simulink model "OFDM0010"  (Simulink 7.7)
settings: Solver=ode45  StartTime=0.0  StopTime=0.08  RelTol=1e-3
undefined symbols (not defined in the file): get, i, rsgenpoly
libraries: dspobslib x46, dspindex x4, commsink2 x3, commutil2 x3, commchan3 x2, commdigbbndam3 x2, dspxfrm3 x2, commblkcod2 x2, commseqgen2 x2, commdigbbndpm3 x2, commrandsrc2 x1, dspsigops x1
Description:
  | This COFDM Simulation by
  | YangZhiguo
  |  .HuNan University at
  |  2011/05/21.
  | The teacher is
  |  xiaoyaoqiang !
  | Thanks to him!
  | This COFDM Simulation simulate Coded OFDM using
  | Reed-Solomon Channel Coding, over wireless multipath
  | fading channel, with 3 us maximal delay spread, 200 Hz
  | Doppler shift.
  | In this simulation I use QPSK, and Training Based
  | Channel Estimation, 11/15 RS Code, 2 Symbol Error
  | Correction
settings Model: Creator=Yangzhiguo  LastModifiedBy=yangzhiguo
settings SolverCC: MaxConsecutiveZCs=10
settings DataIOCC: SignalLoggingName=sigsOut
settings OptimizationCC: InitFltsAndDblsToZero=on
settings DebuggingCC: SaveWithParameterizedLinksMsg=none  SignalResolutionControl=TryResolveAllWithWarning  SolverPrmCheckMsg=none  MultiTaskDSMMsg=warning  MultiTaskCondExecSysMsg=none  StrictBusMsg=None
settings HardwareCC: TargetUnknown=on
settings RTWCC: IncludeERTFirstTime=on

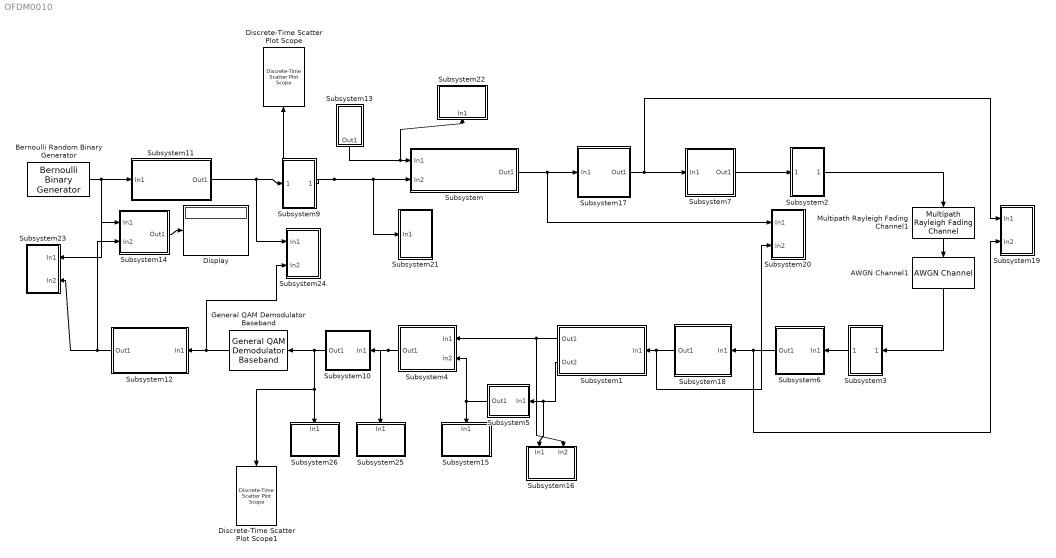
== system OFDM0010 ==
  AWGN Channel1 : commchan3/AWGN Channel  SystemSampleTime=-1  InputProcessing=Inherited (this choice will be removed - see release notes)  seed=32965  noiseMode="Signal to noise ratio  (SNR)"  EbNodB=10  EsNodB=28  SNRdB=-5  bitsPerSym=1  Ps=30/(5.5e5*11/15*2.4)*1.08  Tsym=80e-6  variance=1
  Bernoulli Random Binary Generator : commrandsrc2/Bernoulli Binary Generator  SystemSampleTime=-1  P=[0.5]  seed=9364248  Ts=16e-5/88/2  frameBased=on  sampPerFrame=88  orient=off  outDataType=double
  Discrete-Time Scatter Plot Scope : commsink2/Discrete-Time Scatter Plot Scope  Tag=ScatterPlot  SystemSampleTime=-1  sampPerSymb=1  offsetEye=0  numTraces=40  numNewFrames=40  LineMarkers=.  LineColors=b  fading=on  render=on  AxisGrid=on  xMin=-3.3  xMax=3.315  yMin=-3.3  yMax=3.315  inphaseLabel=In-phase Amplitude  quadratureLabel=Quadrature Amplitude  openScopeAtSimStart=on  FrameNumber=off  FigPos=get(0,'defaultfigureposition');  figTitle=Scatter Plot  numLinesMax=8  block_type_=scatter
  Discrete-Time Scatter Plot Scope1 : commsink2/Discrete-Time Scatter Plot Scope  Tag=ScatterPlot  SystemSampleTime=-1  sampPerSymb=1  offsetEye=0  numTraces=40  numNewFrames=40  LineMarkers=.  LineColors=b  fading=on  render=on  AxisGrid=on  xMin=-3.3  xMax=3.315  yMin=-3.3  yMax=3.315  inphaseLabel=In-phase Amplitude  quadratureLabel=Quadrature Amplitude  openScopeAtSimStart=on  FrameNumber=off  FigPos=get(0,'defaultfigureposition');  figTitle=Scatter Plot  numLinesMax=8  block_type_=scatter
  Display : Display
  General QAM Demodulator Baseband : commdigbbndam3/General QAM Demodulator Baseband  SigCon=[exp(2*pi*i*[0:15]/16)]  OutType=Bit  DecType=Hard decision  VarSource=Dialog  Variance=1  outDtypeBit=Inherit via internal rule  outDtype=Inherit via internal rule  roundingMode=Floor  overflowMode=Wrap  sigConstWordLen=16  accum1WordLen=32  accum1FracLen=30  prodInWordLen=32  prodInFracLen=30  prodOutWordLen=32  prodOutFracLen=30  accum2WordLen=32  accum2FracLen=30  accum3WordLen=32  accum3FracLen=30  nsiWordLen=32  nsiFracLen=30  invn0WordLen=16  invn0FracLen=8  outputWordLen=32  outputFracLen=30
  Multipath Rayleigh Fading Channel1 : commchan3/Multipath Rayleigh Fading Channel  SystemSampleTime=-1  maxDopplerShift=40  spectrumType=Jakes  sigmaGaussian=1/sqrt(2)  coeffRounded=[1 -1.72 0.785]  freqMinMaxRJakes=[0 1]  freqMinMaxAJakes=[0 1]  sigmaGaussian1=1/sqrt(2)  sigmaGaussian2=1/sqrt(2)  centerFreqGaussian1=0.0  centerFreqGaussian2=0.0  gainGaussian1=0.5  gainGaussian2=0.5  coeffBell=9  dopplerSpectrum=doppler.jakes  pathDelays=[0 2e-6]  avgPathGaindB=[0 -12]  normalizePathGains=on  seed=73  enableProbe=0  openVisAtStart=off  outPathGains=off  outDelay=off
  Subsystem : Subsystem
      mask Display: disp('OFDM Baseband\nModulator\ndan\nAdd Cyclic Prefix')
  Subsystem1 : Subsystem
      mask Display: disp('OFDM Baseband\nDemodulator\ndan \nRemove Cyclic prefix')
  Subsystem10 : Subsystem
      mask Display: disp('Remove\nZero')
  Subsystem11 : Subsystem
      mask Display: disp('RS(15,11) Encoder')
  Subsystem12 : Subsystem
      mask Display: disp('RS(15,11) Decoder')
  Subsystem13 : Subsystem
      mask Display: disp('Training')
  Subsystem14 : Subsystem
      mask Display: disp('SER\nCalculation')
  Subsystem15 : Subsystem
  Subsystem16 : Subsystem
  Subsystem17 : Subsystem
      mask Display: disp('Add\nCyclic Prefix')
  Subsystem18 : Subsystem
      mask Display: disp('Remove\nCyclic Prefix')
  Subsystem19 : Subsystem
  Subsystem2 : Subsystem
      mask Display: disp('P/S')
  Subsystem20 : Subsystem
  Subsystem21 : Subsystem
  Subsystem22 : Subsystem
  Subsystem23 : Subsystem
  Subsystem24 : Subsystem
  Subsystem25 : Subsystem
  Subsystem26 : Subsystem
  Subsystem3 : Subsystem
      mask Display: disp('S/P')
  Subsystem4 : Subsystem
      mask Display: disp('Channel\nCompensation')
  Subsystem5 : Subsystem
      mask Display: disp('Channel\nEstimator')
  Subsystem6 : Subsystem
      mask Display: disp('Training\nSeparation')
  Subsystem7 : Subsystem
      mask Display: disp('Training\nInsertion')
  Subsystem9 : Subsystem
      mask Display: disp('16QAM')
  wires:
  Bernoulli Random Binary Generator/1 -> Subsystem14/1(In1), Subsystem11/1(In1), Subsystem23/1(In1)
  Subsystem9/1(Out1) -> Subsystem/2(In2), Subsystem21/1(In1), Discrete-Time Scatter Plot Scope/1
  Subsystem13/1(Out1) -> Subsystem/1(In1), Subsystem22/1(In1)
  Subsystem12/1(Out1) -> Subsystem14/2(In2), Subsystem23/2(In2)
  Subsystem/1(Out1) -> Subsystem17/1(In1), Subsystem20/1(In1)
  Subsystem7/1(Out1) -> Subsystem2/1(In1)
  Subsystem6/1(Out1) -> Subsystem18/1(In1), Subsystem19/2(In2)
  Subsystem14/1(Out1) -> Display/1
  Subsystem3/1(Out1) -> Subsystem6/1(In1)
  Subsystem2/1(Out1) -> Multipath Rayleigh Fading Channel1/1
  Subsystem10/1(Out1) -> Subsystem26/1(In1), Discrete-Time Scatter Plot Scope1/1, General QAM Demodulator Baseband/1
  Multipath Rayleigh Fading Channel1/1 -> AWGN Channel1/1
  AWGN Channel1/1 -> Subsystem3/1(In1)
  Subsystem4/1(Out1) -> Subsystem10/1(In1), Subsystem25/1(In1)
  Subsystem1/1(Out1) -> Subsystem4/1(In1), Subsystem16/2(In2)
  Subsystem5/1(Out1) -> Subsystem4/2(In2), Subsystem15/1(In1)
  Subsystem1/2(Out2) -> Subsystem5/1(In1), Subsystem16/1(In1)
  Subsystem17/1(Out1) -> Subsystem7/1(In1), Subsystem19/1(In1)
  Subsystem18/1(Out1) -> Subsystem1/1(In1), Subsystem20/2(In2)
  General QAM Demodulator Baseband/1 -> Subsystem12/1(In1), Subsystem24/2(In2)
  Subsystem11/1(Out1) -> Subsystem24/1(In1), Subsystem9/1(In1)

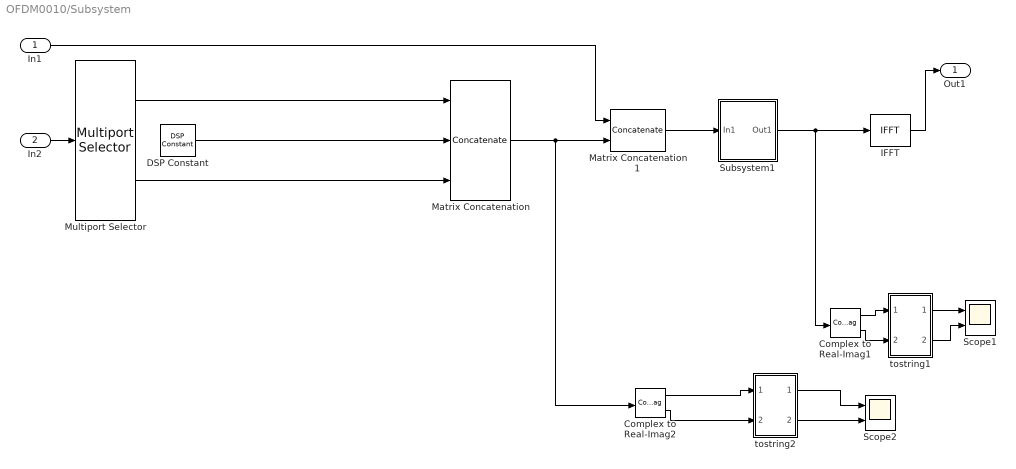
== system OFDM0010/Subsystem ==
  In1 : Inport
  In2 : Inport  Port=2
  Complex to Real-Imag1 : ComplexToRealImag
  Complex to Real-Imag2 : ComplexToRealImag
  DSP Constant : dspobslib/DSP Constant  SystemSampleTime=-1  Value=0  SampleMode=Discrete  discreteOutput=Frame-based  continuousOutput=Sample-based  sampTime=16e-5/2  framePeriod=16e-5/2  dataType=Inherit from 'Constant value'  isSigned=on  wordLen=16  udDataType=sfix(16)  fracBitsMode=Best precision  numFracBits=15  InterpretAs1D=off  Ts=16e-5/2  FramebasedOutput=on
  IFFT : dspxfrm3/IFFT  CompMethod=Table lookup  TableOpt=HYBRID  TableOptActive=Speed  BitRevOrder=off  cs_in=off  SkipNorm=on  InheritFFTLength=on  FFTLength=64  mode=Real  outSamplingMode=Frame based  RowConvenienceOn=on  firstCoeffDataTypeStr=Inherit: Same word length as input  firstCoeffLastDataTypeStr=Inherit: Same word length as input  outputMin=[]  outputMax=[]  roundingMode=Floor  overflowMode=off
  Matrix Concatenation : Concatenate  NumInputs=3  Mode=Multidimensional array
  Matrix Concatenation1 : Concatenate  Mode=Multidimensional array  ConcatenateDimension=2
  Multiport Selector : dspindex/Multiport Selector  rowsOrCols=Rows  idxCellArray={1:15,16:30}  idxErrMode=Clip Index
  Scope1 : Scope  NumInputPorts=2
      settings: YMin=-5~-5  YMax=5~5  SaveName=ScopeData5
  Scope2 : Scope  NumInputPorts=2
      settings: YMin=-5~-5  YMax=5~5  SaveName=ScopeData6
  Subsystem1 : Subsystem
      mask Display: disp('Zero Pad')
  tostring1 : Subsystem
  tostring2 : Subsystem
  Out1 : Outport
  wires:
  IFFT/1 -> Out1/1
  Multiport Selector/1 -> Matrix Concatenation/1
  Multiport Selector/2 -> Matrix Concatenation/3
  DSP Constant/1 -> Matrix Concatenation/2
  Subsystem1/1(Out1) -> IFFT/1, Complex to Real-Imag1/1
  In2/1 -> Multiport Selector/1
  Matrix Concatenation1/1 -> Subsystem1/1(In1)
  Matrix Concatenation/1 -> Matrix Concatenation1/2, Complex to Real-Imag2/1
  In1/1 -> Matrix Concatenation1/1
  Complex to Real-Imag1/1 -> tostring1/1(In1)
  Complex to Real-Imag1/2 -> tostring1/2(In2)
  tostring1/1(Out1) -> Scope1/1
  tostring1/2(Out2) -> Scope1/2
  Complex to Real-Imag2/1 -> tostring2/1(In1)
  Complex to Real-Imag2/2 -> tostring2/2(In2)
  tostring2/1(Out1) -> Scope2/1
  tostring2/2(Out2) -> Scope2/2

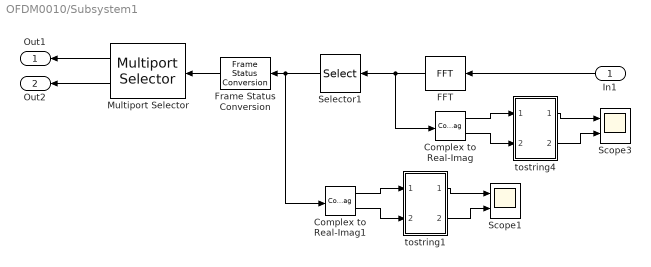
== system OFDM0010/Subsystem1 ==
  In1 : Inport
  Complex to Real-Imag : ComplexToRealImag
  Complex to Real-Imag1 : ComplexToRealImag
  FFT : dspxfrm3/FFT  CompMethod=Table lookup  TableOpt=HYBRID  TableOptActive=Speed  BitRevOrder=off  InheritFFTLength=on  FFTLength=64  RowConvenienceOn=on  SkipNorm=off  firstCoeffDataTypeStr=Inherit: Same word length as input  firstCoeffLastDataTypeStr=Inherit: Same word length as input  outputMin=[]  outputMax=[]  roundingMode=Floor  overflowMode=off
  Frame Status Conversion : dspobslib/Frame Status Conversion  SystemSampleTime=-1  growRefPort=off  outframe=Frame-based
  Multiport Selector : dspindex/Multiport Selector  rowsOrCols=Columns  idxCellArray={1,2}  idxErrMode=Clip Index
  Scope1 : Scope  NumInputPorts=2
      settings: YMin=-5~-5  YMax=5~5  SaveName=ScopeData9
  Scope3 : Scope  NumInputPorts=2
      settings: YMin=-5~-5  YMax=5~5  SaveName=ScopeData8
  Selector1 : Selector  NumberOfDimensions=2  InputPortWidth=64  IndexOptions=Index vector (dialog),Select all  Indices=[50:64,1:16],-1  OutputSizes=1
  tostring1 : Subsystem
  tostring4 : Subsystem
  Out1 : Outport
  Out2 : Outport  Port=2
  wires:
  FFT/1 -> Selector1/1, Complex to Real-Imag/1
  Selector1/1 -> Frame Status Conversion/1, Complex to Real-Imag1/1
  In1/1 -> FFT/1
  Frame Status Conversion/1 -> Multiport Selector/1
  Multiport Selector/1 -> Out1/1
  Multiport Selector/2 -> Out2/1
  Complex to Real-Imag/1 -> tostring4/1(In1)
  Complex to Real-Imag/2 -> tostring4/2(In2)
  tostring4/1(Out1) -> Scope3/1
  tostring4/2(Out2) -> Scope3/2
  Complex to Real-Imag1/1 -> tostring1/1(In1)
  Complex to Real-Imag1/2 -> tostring1/2(In2)
  tostring1/1(Out1) -> Scope1/1
  tostring1/2(Out2) -> Scope1/2

== system OFDM0010/Subsystem10 ==
  In1 : Inport
  Selector2 : Selector  NumberOfDimensions=2  InputPortWidth=31  IndexOptions=Index vector (dialog),Select all  Indices=[1:15,17:31],-1  OutputSizes=1
  Out1 : Outport
  wires:
  Selector2/1 -> Out1/1
  In1/1 -> Selector2/1

== system OFDM0010/Subsystem11 ==
  In1 : Inport
  Binary-Input RS Encoder : commblkcod2/Binary-Input RS Encoder  SystemSampleTime=-1  n=15  k=11  specPrimPoly=off  prPoly=[1 0 1 1]  specGenPoly=off  genPoly=rsgenpoly(7,3)  specPuncture=off  punctVec=[ones(2,1); zeros(2,1)]  outDType=Same as input
  Out1 : Outport
  wires:
  In1/1 -> Binary-Input RS Encoder/1
  Binary-Input RS Encoder/1 -> Out1/1

== system OFDM0010/Subsystem12 ==
  In1 : Inport
  Binary-Output RS Decoder : commblkcod2/Binary-Output RS Decoder  SystemSampleTime=-1  n=15  k=11  specPrimPoly=off  prPoly=[1 0 1 1]  specGenPoly=off  genPoly=rsgenpoly(7,3)  specPuncture=off  punctVec=[ones(2,1); zeros(2,1)]  specErasurePort=off  showNumErr=on  outDType=Same as input
  Terminator : Terminator
  Out1 : Outport
  wires:
  Binary-Output RS Decoder/2 -> Terminator/1
  Binary-Output RS Decoder/1 -> Out1/1
  In1/1 -> Binary-Output RS Decoder/1

== system OFDM0010/Subsystem13 ==
  PN Sequence Generator : commseqgen2/PN Sequence Generator  poly=[1 0 0 0 0 1 1]  ini_sta=[0 0 0 0 0 1]  outBitMaskSource=Dialog parameter  shift=0  outVarSiz=off  maxOutSizeMode=Dialog parameter  maxOutSize=[10 1]  Ts=16e-5/2/31  frameBased=on  sampPerFrame=31  reset=off  bitPackedOutputs=off  outDataType=double  numPackedBits=8  bitPackDataSigned=off  bitPackedOutDType=double
  Unipolar to Bipolar Converter : commutil2/Unipolar to Bipolar Converter  SystemSampleTime=-1  M=2  polarity=Positive  dataType=Inherit via internal rule
  Out1 : Outport
  wires:
  PN Sequence Generator/1 -> Unipolar to Bipolar Converter/1
  Unipolar to Bipolar Converter/1 -> Out1/1

== system OFDM0010/Subsystem14 ==
  In1 : Inport
  In2 : Inport  Port=2
  Error Rate Calculation : commsink2/Error Rate Calculation  N=44  st_delay=0  cp_mode=Entire frame  subframe=[]  PMode=Port  WsName=ErrorVec  RsMode2=off  stop=off  numErr=inf  maxBits=2e4
  QPSK Modulator Baseband : commdigbbndpm3/QPSK Modulator Baseband  SystemSampleTime=-1  InType=Bit  Enc=Binary  Ph=pi/4  outDtype=double  outWordLen=16  outUDDataType=sfix(16)  outFracLenMode=Best precision  outFracLen=15
  QPSK Modulator Baseband1 : commdigbbndpm3/QPSK Modulator Baseband  SystemSampleTime=-1  InType=Bit  Enc=Binary  Ph=pi/4  outDtype=double  outWordLen=16  outUDDataType=sfix(16)  outFracLenMode=Best precision  outFracLen=15
  Out1 : Outport
  wires:
  QPSK Modulator Baseband/1 -> Error Rate Calculation/1
  QPSK Modulator Baseband1/1 -> Error Rate Calculation/2
  In1/1 -> QPSK Modulator Baseband/1
  Error Rate Calculation/1 -> Out1/1
  In2/1 -> QPSK Modulator Baseband1/1

== system OFDM0010/Subsystem15 ==
  In1 : Inport
  Complex to Real-Imag7 : ComplexToRealImag
  Scope7 : Scope  NumInputPorts=2
      settings: YMin=-5~-5  YMax=5~5  SaveName=ScopeData11
  tostring9 : Subsystem
  wires:
  Complex to Real-Imag7/1 -> tostring9/1(In1)
  Complex to Real-Imag7/2 -> tostring9/2(In2)
  tostring9/1(Out1) -> Scope7/1
  tostring9/2(Out2) -> Scope7/2
  In1/1 -> Complex to Real-Imag7/1

== system OFDM0010/Subsystem16 ==
  In1 : Inport
  In2 : Inport  Port=2
  Complex to Real-Imag5 : ComplexToRealImag
  Complex to Real-Imag6 : ComplexToRealImag
  Scope6 : Scope  NumInputPorts=4
      settings: YMin=-5~-5~-5~-5  YMax=5~5~5~5  SaveName=ScopeData10
  tostring8 : Subsystem
  wires:
  tostring8/1(Out1) -> Scope6/1
  tostring8/2(Out2) -> Scope6/2
  Complex to Real-Imag5/1 -> tostring8/1(In1)
  Complex to Real-Imag5/2 -> tostring8/2(In2)
  Complex to Real-Imag6/1 -> tostring8/3(In3)
  Complex to Real-Imag6/2 -> tostring8/4(In4)
  tostring8/3(Out3) -> Scope6/3
  tostring8/4(Out4) -> Scope6/4
  In1/1 -> Complex to Real-Imag5/1
  In2/1 -> Complex to Real-Imag6/1

== system OFDM0010/Subsystem17 ==
  In1 : Inport
  Selector3 : Selector  NumberOfDimensions=2  InputPortWidth=64  IndexOptions=Index vector (dialog),Select all  Indices=[39:64,1:64],-1  OutputSizes=1
  Out1 : Outport
  wires:
  Selector3/1 -> Out1/1
  In1/1 -> Selector3/1

== system OFDM0010/Subsystem18 ==
  In1 : Inport
  Selector4 : Selector  NumberOfDimensions=2  InputPortWidth=78  IndexOptions=Index vector (dialog),Select all  Indices=[27:90],-1  OutputSizes=1
  Out1 : Outport
  wires:
  Selector4/1 -> Out1/1
  In1/1 -> Selector4/1

== system OFDM0010/Subsystem19 ==
  In1 : Inport
  In2 : Inport  Port=2
  Complex to Real-Imag1 : ComplexToRealImag
  Complex to Real-Imag2 : ComplexToRealImag
  Scope4 : Scope  NumInputPorts=4
      settings: YMin=-5~-5~-5~-5  YMax=5~5~5~5  SaveName=ScopeData7
  tostring5 : Subsystem
  tostring6 : Subsystem
  wires:
  Complex to Real-Imag1/1 -> tostring5/1(In1)
  Complex to Real-Imag1/2 -> tostring5/2(In2)
  tostring5/1(Out1) -> Scope4/1
  Complex to Real-Imag2/1 -> tostring6/1(In1)
  Complex to Real-Imag2/2 -> tostring6/2(In2)
  tostring6/1(Out1) -> Scope4/2
  tostring5/2(Out2) -> Scope4/3
  tostring6/2(Out2) -> Scope4/4
  In1/1 -> Complex to Real-Imag1/1
  In2/1 -> Complex to Real-Imag2/1

== system OFDM0010/Subsystem2 ==
  In1 : Inport
  Unbuffer3 : Unbuffer
  Out1 : Outport
  wires:
  In1/1 -> Unbuffer3/1
  Unbuffer3/1 -> Out1/1

== system OFDM0010/Subsystem20 ==
  In1 : Inport
  In2 : Inport  Port=2
  Complex to Real-Imag3 : ComplexToRealImag
  Complex to Real-Imag4 : ComplexToRealImag
  Scope5 : Scope  NumInputPorts=4
      settings: YMin=-5~-5~-5~-5  YMax=5~5~5~5  SaveName=ScopeData4
  tostring7 : Subsystem
  wires:
  Complex to Real-Imag3/1 -> tostring7/1(In1)
  Complex to Real-Imag3/2 -> tostring7/2(In2)
  tostring7/1(Out1) -> Scope5/1
  Complex to Real-Imag4/1 -> tostring7/3(In3)
  Complex to Real-Imag4/2 -> tostring7/4(In4)
  tostring7/3(Out3) -> Scope5/2
  tostring7/2(Out2) -> Scope5/3
  tostring7/4(Out4) -> Scope5/4
  In1/1 -> Complex to Real-Imag3/1
  In2/1 -> Complex to Real-Imag4/1

== system OFDM0010/Subsystem21 ==
  In1 : Inport
  Complex to Real-Imag : ComplexToRealImag
  Scope3 : Scope  NumInputPorts=2
      settings: YMin=-5~-5  YMax=5~5  SaveName=ScopeData3
  tostring4 : Subsystem
  wires:
  Complex to Real-Imag/1 -> tostring4/1(In1)
  Complex to Real-Imag/2 -> tostring4/2(In2)
  tostring4/1(Out1) -> Scope3/1
  tostring4/2(Out2) -> Scope3/2
  In1/1 -> Complex to Real-Imag/1

== system OFDM0010/Subsystem22 ==
  In1 : Inport
  Scope2 : Scope
      settings: SaveName=ScopeData2
  tostring3 : Subsystem
  wires:
  tostring3/1(Out1) -> Scope2/1
  In1/1 -> tostring3/1(In1)

== system OFDM0010/Subsystem23 ==
  In1 : Inport
  In2 : Inport  Port=2
  Scope : Scope  NumInputPorts=2
      settings: YMin=-5~-5  YMax=5~5
  tostring : Subsystem
  tostring1 : Subsystem
  wires:
  tostring/1(Out1) -> Scope/1
  tostring1/1(Out1) -> Scope/2
  In1/1 -> tostring/1(In1)
  In2/1 -> tostring1/1(In1)

== system OFDM0010/Subsystem24 ==
  In1 : Inport
  In2 : Inport  Port=2
  Scope1 : Scope  NumInputPorts=2
      settings: YMin=-5~-5  YMax=5~5
  tostring2 : Subsystem
  wires:
  tostring2/1(Out1) -> Scope1/1
  tostring2/2(Out2) -> Scope1/2
  In1/1 -> tostring2/1(In1)
  In2/1 -> tostring2/2(In2)

== system OFDM0010/Subsystem25 ==
  In1 : Inport
  Complex to Real-Imag7 : ComplexToRealImag
  Scope7 : Scope  NumInputPorts=2
      settings: YMin=-5~-5  YMax=5~5  SaveName=ScopeData11
  tostring9 : Subsystem
  wires:
  Complex to Real-Imag7/1 -> tostring9/1(In1)
  Complex to Real-Imag7/2 -> tostring9/2(In2)
  tostring9/1(Out1) -> Scope7/1
  tostring9/2(Out2) -> Scope7/2
  In1/1 -> Complex to Real-Imag7/1

== system OFDM0010/Subsystem26 ==
  In1 : Inport
  Complex to Real-Imag7 : ComplexToRealImag
  Scope7 : Scope  NumInputPorts=2
      settings: YMin=-5~-5  YMax=5~5  SaveName=ScopeData11
  tostring9 : Subsystem
  wires:
  Complex to Real-Imag7/1 -> tostring9/1(In1)
  Complex to Real-Imag7/2 -> tostring9/2(In2)
  tostring9/1(Out1) -> Scope7/1
  tostring9/2(Out2) -> Scope7/2
  In1/1 -> Complex to Real-Imag7/1

== system OFDM0010/Subsystem3 ==
  In1 : Inport
  Buffer : Buffer  N=180
  Out1 : Outport
  wires:
  In1/1 -> Buffer/1
  Buffer/1 -> Out1/1

== system OFDM0010/Subsystem4 ==
  In1 : Inport
  In2 : Inport  Port=2
  Frame Status Conversion5 : dspobslib/Frame Status Conversion  SystemSampleTime=-1  growRefPort=off  outframe=Frame-based
  Product : Product  SaturateOnIntegerOverflow=on  OutDataTypeStr=Inherit: Same as first input
  Out1 : Outport
  wires:
  Frame Status Conversion5/1 -> Out1/1
  In2/1 -> Product/1
  Product/1 -> Frame Status Conversion5/1
  In1/1 -> Product/2

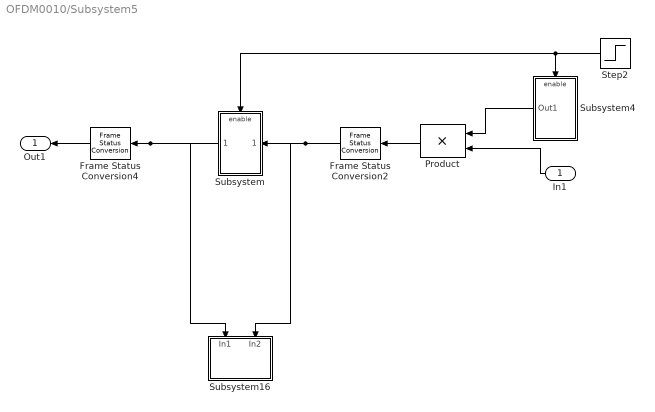
== system OFDM0010/Subsystem5 ==
  In1 : Inport
  Frame Status Conversion2 : dspobslib/Frame Status Conversion  SystemSampleTime=-1  growRefPort=off  outframe=Frame-based
  Frame Status Conversion4 : dspobslib/Frame Status Conversion  SystemSampleTime=-1  growRefPort=off  outframe=Frame-based
  Product : Product  SaturateOnIntegerOverflow=on  OutDataTypeStr=Inherit: Same as first input
  Step2 : Step  Time=16e-5/2  SampleTime=16e-5/2
  Subsystem : Subsystem
  Subsystem16 : Subsystem
  Subsystem4 : Subsystem  TreatAsAtomicUnit=on
  Out1 : Outport
  wires:
  Step2/1 -> Subsystem4/Enable, Subsystem/Enable
  Subsystem4/1(Out1) -> Product/1
  Product/1 -> Frame Status Conversion2/1
  Frame Status Conversion2/1 -> Subsystem/1(In1), Subsystem16/2(In2)
  Frame Status Conversion4/1 -> Out1/1
  In1/1 -> Product/2
  Subsystem/1(Out1) -> Frame Status Conversion4/1, Subsystem16/1(In1)

== system OFDM0010/Subsystem6 ==
  In1 : Inport
  Matrix Concatenation1 : Concatenate  Mode=Multidimensional array  ConcatenateDimension=2
  Multiport Selector1 : dspindex/Multiport Selector  rowsOrCols=Rows  idxCellArray={91:180,1:90}  idxErrMode=Clip Index
  Out1 : Outport
  wires:
  Multiport Selector1/2 -> Matrix Concatenation1/2
  Multiport Selector1/1 -> Matrix Concatenation1/1
  In1/1 -> Multiport Selector1/1
  Matrix Concatenation1/1 -> Out1/1

== system OFDM0010/Subsystem7 ==
  In1 : Inport
  Frame Status Conversion : dspobslib/Frame Status Conversion  SystemSampleTime=-1  growRefPort=off  outframe=Frame-based
  Matrix Concatenation : Concatenate  Mode=Multidimensional array
  Multiport Selector : dspindex/Multiport Selector  rowsOrCols=Columns  idxCellArray={1,2}  idxErrMode=Clip Index
  Out1 : Outport
  wires:
  Multiport Selector/1 -> Matrix Concatenation/1
  Multiport Selector/2 -> Matrix Concatenation/2
  Matrix Concatenation/1 -> Frame Status Conversion/1
  In1/1 -> Multiport Selector/1
  Frame Status Conversion/1 -> Out1/1

== system OFDM0010/Subsystem9 ==
  In1 : Inport
  Bit to Integer Converter : commutil2/Bit to Integer Converter  nbits=4  bitOrder=MSB first  signedOutputValues=Unsigned  outDtype=double  outDtypeSigned=Inherit via internal rule
  General QAM Modulator Baseband : commdigbbndam3/General QAM Modulator Baseband  SigCon=[exp(2*pi*i*[0:15]/16)]  outDtype=double  outWordLen=16  outUDDataType=sfix(16)  outFracLenMode=Best precision  outFracLen=15
  Out1 : Outport
  wires:
  Bit to Integer Converter/1 -> General QAM Modulator Baseband/1
  In1/1 -> Bit to Integer Converter/1
  General QAM Modulator Baseband/1 -> Out1/1

== system OFDM0010/Subsystem/Subsystem1 ==
  In1 : Inport
  Selector : Selector  NumberOfDimensions=2  InputPortWidth=64  IndexOptions=Index vector (dialog),Select all  Indices=[16:64,1:15],-1  OutputSizes=1
  Zero Pad : dspsigops/Pad  padAlong=Columns and rows  dimsToPad=1  valSrc=Specify via dialog  padVal=0  spec=Output size  padNumOutRowsSpecMethod=User-specified  numOutRows=64  padNumOutColsSpecMethod=User-specified  numOutCols=2  isVarDimsMode=off  padBeginning=0  padEnd=0  outSizeMode=User-specified  outSize=1  padSigAt=End  trunc_flag=None  roundingMode=Floor  overflowMode=off  truncOrWrapMode=Truncate  wrap_flag=None
  Out1 : Outport
  wires:
  Zero Pad/1 -> Selector/1
  In1/1 -> Zero Pad/1
  Selector/1 -> Out1/1

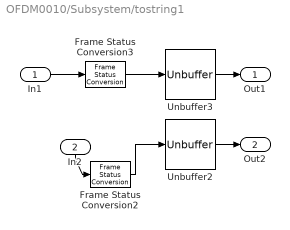
== system OFDM0010/Subsystem/tostring1 ==
  In1 : Inport
  In2 : Inport  Port=2
  Frame Status Conversion2 : dspobslib/Frame Status Conversion  SystemSampleTime=-1  growRefPort=off  outframe=Sample-based
  Frame Status Conversion3 : dspobslib/Frame Status Conversion  SystemSampleTime=-1  growRefPort=off  outframe=Sample-based
  Unbuffer2 : Unbuffer  SampleBasedProcessing=Same as frame based
  Unbuffer3 : Unbuffer  SampleBasedProcessing=Same as frame based
  Out1 : Outport
  Out2 : Outport  Port=2
  wires:
  Frame Status Conversion3/1 -> Unbuffer3/1
  Frame Status Conversion2/1 -> Unbuffer2/1
  In1/1 -> Frame Status Conversion3/1
  In2/1 -> Frame Status Conversion2/1
  Unbuffer3/1 -> Out1/1
  Unbuffer2/1 -> Out2/1

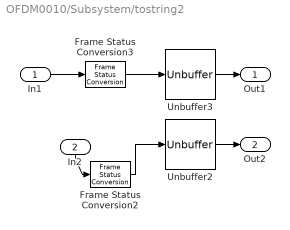
== system OFDM0010/Subsystem/tostring2 ==
  In1 : Inport
  In2 : Inport  Port=2
  Frame Status Conversion2 : dspobslib/Frame Status Conversion  SystemSampleTime=-1  growRefPort=off  outframe=Sample-based
  Frame Status Conversion3 : dspobslib/Frame Status Conversion  SystemSampleTime=-1  growRefPort=off  outframe=Sample-based
  Unbuffer2 : Unbuffer  SampleBasedProcessing=Same as frame based
  Unbuffer3 : Unbuffer  SampleBasedProcessing=Same as frame based
  Out1 : Outport
  Out2 : Outport  Port=2
  wires:
  Frame Status Conversion3/1 -> Unbuffer3/1
  Frame Status Conversion2/1 -> Unbuffer2/1
  In1/1 -> Frame Status Conversion3/1
  In2/1 -> Frame Status Conversion2/1
  Unbuffer3/1 -> Out1/1
  Unbuffer2/1 -> Out2/1

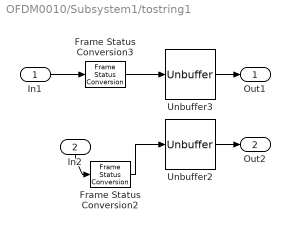
== system OFDM0010/Subsystem1/tostring1 ==
  In1 : Inport
  In2 : Inport  Port=2
  Frame Status Conversion2 : dspobslib/Frame Status Conversion  SystemSampleTime=-1  growRefPort=off  outframe=Sample-based
  Frame Status Conversion3 : dspobslib/Frame Status Conversion  SystemSampleTime=-1  growRefPort=off  outframe=Sample-based
  Unbuffer2 : Unbuffer  SampleBasedProcessing=Same as frame based
  Unbuffer3 : Unbuffer  SampleBasedProcessing=Same as frame based
  Out1 : Outport
  Out2 : Outport  Port=2
  wires:
  Frame Status Conversion3/1 -> Unbuffer3/1
  Frame Status Conversion2/1 -> Unbuffer2/1
  In1/1 -> Frame Status Conversion3/1
  In2/1 -> Frame Status Conversion2/1
  Unbuffer3/1 -> Out1/1
  Unbuffer2/1 -> Out2/1

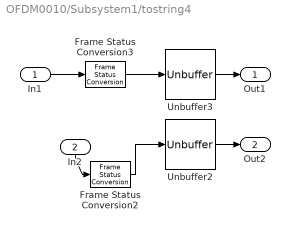
== system OFDM0010/Subsystem1/tostring4 ==
  In1 : Inport
  In2 : Inport  Port=2
  Frame Status Conversion2 : dspobslib/Frame Status Conversion  SystemSampleTime=-1  growRefPort=off  outframe=Sample-based
  Frame Status Conversion3 : dspobslib/Frame Status Conversion  SystemSampleTime=-1  growRefPort=off  outframe=Sample-based
  Unbuffer2 : Unbuffer  SampleBasedProcessing=Same as frame based
  Unbuffer3 : Unbuffer  SampleBasedProcessing=Same as frame based
  Out1 : Outport
  Out2 : Outport  Port=2
  wires:
  Frame Status Conversion3/1 -> Unbuffer3/1
  Frame Status Conversion2/1 -> Unbuffer2/1
  In1/1 -> Frame Status Conversion3/1
  In2/1 -> Frame Status Conversion2/1
  Unbuffer3/1 -> Out1/1
  Unbuffer2/1 -> Out2/1

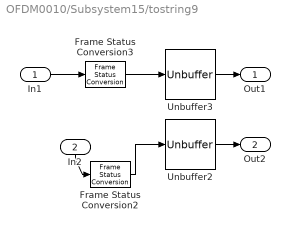
== system OFDM0010/Subsystem15/tostring9 ==
  In1 : Inport
  In2 : Inport  Port=2
  Frame Status Conversion2 : dspobslib/Frame Status Conversion  SystemSampleTime=-1  growRefPort=off  outframe=Sample-based
  Frame Status Conversion3 : dspobslib/Frame Status Conversion  SystemSampleTime=-1  growRefPort=off  outframe=Sample-based
  Unbuffer2 : Unbuffer  SampleBasedProcessing=Same as frame based
  Unbuffer3 : Unbuffer  SampleBasedProcessing=Same as frame based
  Out1 : Outport
  Out2 : Outport  Port=2
  wires:
  Frame Status Conversion3/1 -> Unbuffer3/1
  Frame Status Conversion2/1 -> Unbuffer2/1
  In1/1 -> Frame Status Conversion3/1
  In2/1 -> Frame Status Conversion2/1
  Unbuffer3/1 -> Out1/1
  Unbuffer2/1 -> Out2/1

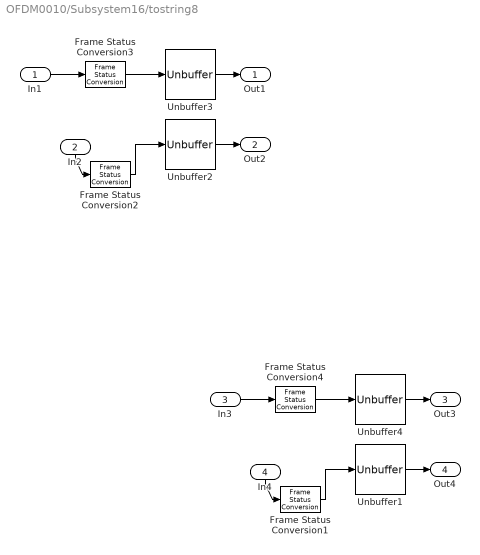
== system OFDM0010/Subsystem16/tostring8 ==
  In1 : Inport
  In2 : Inport  Port=2
  In3 : Inport  Port=3
  In4 : Inport  Port=4
  Frame Status Conversion{1..4} (4 alike) : dspobslib/Frame Status Conversion  SystemSampleTime=-1  growRefPort=off  outframe=Sample-based
  Unbuffer{1..4} (4 alike) : Unbuffer  SampleBasedProcessing=Same as frame based
  Out1 : Outport
  Out2 : Outport  Port=2
  Out3 : Outport  Port=3
  Out4 : Outport  Port=4
  wires:
  Frame Status Conversion3/1 -> Unbuffer3/1
  Frame Status Conversion2/1 -> Unbuffer2/1
  In1/1 -> Frame Status Conversion3/1
  In2/1 -> Frame Status Conversion2/1
  Unbuffer3/1 -> Out1/1
  Unbuffer2/1 -> Out2/1
  Frame Status Conversion4/1 -> Unbuffer4/1
  Frame Status Conversion1/1 -> Unbuffer1/1
  In3/1 -> Frame Status Conversion4/1
  In4/1 -> Frame Status Conversion1/1
  Unbuffer4/1 -> Out3/1
  Unbuffer1/1 -> Out4/1

== system OFDM0010/Subsystem19/tostring5 ==
  In1 : Inport
  In2 : Inport  Port=2
  Frame Status Conversion2 : dspobslib/Frame Status Conversion  SystemSampleTime=-1  growRefPort=off  outframe=Sample-based
  Frame Status Conversion3 : dspobslib/Frame Status Conversion  SystemSampleTime=-1  growRefPort=off  outframe=Sample-based
  Unbuffer2 : Unbuffer  SampleBasedProcessing=Same as frame based
  Unbuffer3 : Unbuffer  SampleBasedProcessing=Same as frame based
  Out1 : Outport
  Out2 : Outport  Port=2
  wires:
  Frame Status Conversion3/1 -> Unbuffer3/1
  Frame Status Conversion2/1 -> Unbuffer2/1
  In1/1 -> Frame Status Conversion3/1
  In2/1 -> Frame Status Conversion2/1
  Unbuffer3/1 -> Out1/1
  Unbuffer2/1 -> Out2/1

== system OFDM0010/Subsystem19/tostring6 ==
  In1 : Inport
  In2 : Inport  Port=2
  Frame Status Conversion2 : dspobslib/Frame Status Conversion  SystemSampleTime=-1  growRefPort=off  outframe=Sample-based
  Frame Status Conversion3 : dspobslib/Frame Status Conversion  SystemSampleTime=-1  growRefPort=off  outframe=Sample-based
  Unbuffer2 : Unbuffer  SampleBasedProcessing=Same as frame based
  Unbuffer3 : Unbuffer  SampleBasedProcessing=Same as frame based
  Out1 : Outport
  Out2 : Outport  Port=2
  wires:
  Frame Status Conversion3/1 -> Unbuffer3/1
  Frame Status Conversion2/1 -> Unbuffer2/1
  In1/1 -> Frame Status Conversion3/1
  In2/1 -> Frame Status Conversion2/1
  Unbuffer3/1 -> Out1/1
  Unbuffer2/1 -> Out2/1

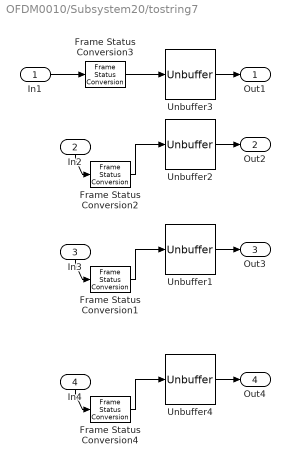
== system OFDM0010/Subsystem20/tostring7 ==
  In1 : Inport
  In2 : Inport  Port=2
  In3 : Inport  Port=3
  In4 : Inport  Port=4
  Frame Status Conversion{1..4} (4 alike) : dspobslib/Frame Status Conversion  SystemSampleTime=-1  growRefPort=off  outframe=Sample-based
  Unbuffer{1..4} (4 alike) : Unbuffer  SampleBasedProcessing=Same as frame based
  Out1 : Outport
  Out2 : Outport  Port=2
  Out3 : Outport  Port=3
  Out4 : Outport  Port=4
  wires:
  Frame Status Conversion3/1 -> Unbuffer3/1
  Frame Status Conversion2/1 -> Unbuffer2/1
  In1/1 -> Frame Status Conversion3/1
  In2/1 -> Frame Status Conversion2/1
  Unbuffer3/1 -> Out1/1
  Unbuffer2/1 -> Out2/1
  Frame Status Conversion1/1 -> Unbuffer1/1
  In3/1 -> Frame Status Conversion1/1
  Unbuffer1/1 -> Out3/1
  Frame Status Conversion4/1 -> Unbuffer4/1
  In4/1 -> Frame Status Conversion4/1
  Unbuffer4/1 -> Out4/1

== system OFDM0010/Subsystem21/tostring4 ==
  In1 : Inport
  In2 : Inport  Port=2
  Frame Status Conversion2 : dspobslib/Frame Status Conversion  SystemSampleTime=-1  growRefPort=off  outframe=Sample-based
  Frame Status Conversion3 : dspobslib/Frame Status Conversion  SystemSampleTime=-1  growRefPort=off  outframe=Sample-based
  Unbuffer2 : Unbuffer  SampleBasedProcessing=Same as frame based
  Unbuffer3 : Unbuffer  SampleBasedProcessing=Same as frame based
  Out1 : Outport
  Out2 : Outport  Port=2
  wires:
  Frame Status Conversion3/1 -> Unbuffer3/1
  Frame Status Conversion2/1 -> Unbuffer2/1
  In1/1 -> Frame Status Conversion3/1
  In2/1 -> Frame Status Conversion2/1
  Unbuffer3/1 -> Out1/1
  Unbuffer2/1 -> Out2/1

== system OFDM0010/Subsystem22/tostring3 ==
  In1 : Inport
  Frame Status Conversion1 : dspobslib/Frame Status Conversion  SystemSampleTime=-1  growRefPort=off  outframe=Sample-based
  Unbuffer1 : Unbuffer  SampleBasedProcessing=Same as frame based
  Out1 : Outport
  wires:
  Frame Status Conversion1/1 -> Unbuffer1/1
  In1/1 -> Frame Status Conversion1/1
  Unbuffer1/1 -> Out1/1

== system OFDM0010/Subsystem23/tostring ==
  In1 : Inport
  Frame Status Conversion5 : dspobslib/Frame Status Conversion  SystemSampleTime=-1  growRefPort=off  outframe=Sample-based
  Unbuffer : Unbuffer  SampleBasedProcessing=Same as frame based
  Out1 : Outport
  wires:
  Frame Status Conversion5/1 -> Unbuffer/1
  In1/1 -> Frame Status Conversion5/1
  Unbuffer/1 -> Out1/1

== system OFDM0010/Subsystem23/tostring1 ==
  In1 : Inport
  Frame Status Conversion1 : dspobslib/Frame Status Conversion  SystemSampleTime=-1  growRefPort=off  outframe=Sample-based
  Unbuffer1 : Unbuffer  SampleBasedProcessing=Same as frame based
  Out1 : Outport
  wires:
  Frame Status Conversion1/1 -> Unbuffer1/1
  In1/1 -> Frame Status Conversion1/1
  Unbuffer1/1 -> Out1/1

== system OFDM0010/Subsystem24/tostring2 ==
  In1 : Inport
  In2 : Inport  Port=2
  Frame Status Conversion2 : dspobslib/Frame Status Conversion  SystemSampleTime=-1  growRefPort=off  outframe=Sample-based
  Frame Status Conversion3 : dspobslib/Frame Status Conversion  SystemSampleTime=-1  growRefPort=off  outframe=Sample-based
  Unbuffer2 : Unbuffer  SampleBasedProcessing=Same as frame based
  Unbuffer3 : Unbuffer  SampleBasedProcessing=Same as frame based
  Out1 : Outport
  Out2 : Outport  Port=2
  wires:
  Frame Status Conversion3/1 -> Unbuffer3/1
  Frame Status Conversion2/1 -> Unbuffer2/1
  In1/1 -> Frame Status Conversion3/1
  In2/1 -> Frame Status Conversion2/1
  Unbuffer3/1 -> Out1/1
  Unbuffer2/1 -> Out2/1

== system OFDM0010/Subsystem25/tostring9 ==
  In1 : Inport
  In2 : Inport  Port=2
  Frame Status Conversion2 : dspobslib/Frame Status Conversion  SystemSampleTime=-1  growRefPort=off  outframe=Sample-based
  Frame Status Conversion3 : dspobslib/Frame Status Conversion  SystemSampleTime=-1  growRefPort=off  outframe=Sample-based
  Unbuffer2 : Unbuffer  SampleBasedProcessing=Same as frame based
  Unbuffer3 : Unbuffer  SampleBasedProcessing=Same as frame based
  Out1 : Outport
  Out2 : Outport  Port=2
  wires:
  Frame Status Conversion3/1 -> Unbuffer3/1
  Frame Status Conversion2/1 -> Unbuffer2/1
  In1/1 -> Frame Status Conversion3/1
  In2/1 -> Frame Status Conversion2/1
  Unbuffer3/1 -> Out1/1
  Unbuffer2/1 -> Out2/1

== system OFDM0010/Subsystem26/tostring9 ==
  In1 : Inport
  In2 : Inport  Port=2
  Frame Status Conversion2 : dspobslib/Frame Status Conversion  SystemSampleTime=-1  growRefPort=off  outframe=Sample-based
  Frame Status Conversion3 : dspobslib/Frame Status Conversion  SystemSampleTime=-1  growRefPort=off  outframe=Sample-based
  Unbuffer2 : Unbuffer  SampleBasedProcessing=Same as frame based
  Unbuffer3 : Unbuffer  SampleBasedProcessing=Same as frame based
  Out1 : Outport
  Out2 : Outport  Port=2
  wires:
  Frame Status Conversion3/1 -> Unbuffer3/1
  Frame Status Conversion2/1 -> Unbuffer2/1
  In1/1 -> Frame Status Conversion3/1
  In2/1 -> Frame Status Conversion2/1
  Unbuffer3/1 -> Out1/1
  Unbuffer2/1 -> Out2/1

== system OFDM0010/Subsystem5/Subsystem ==
  In1 : Inport
  Enable : EnablePort
  Math Function : Math  Operator=reciprocal  SaturateOnIntegerOverflow=on
  Out1 : Outport
  wires:
  In1/1 -> Math Function/1
  Math Function/1 -> Out1/1

== system OFDM0010/Subsystem5/Subsystem16 ==
  In1 : Inport
  In2 : Inport  Port=2
  Complex to Real-Imag5 : ComplexToRealImag
  Complex to Real-Imag6 : ComplexToRealImag
  Scope6 : Scope  NumInputPorts=4
      settings: YMin=-5~-5~-5~-5  YMax=5~5~5~5  SaveName=ScopeData10
  tostring8 : Subsystem
  wires:
  tostring8/1(Out1) -> Scope6/1
  tostring8/2(Out2) -> Scope6/2
  Complex to Real-Imag5/1 -> tostring8/1(In1)
  Complex to Real-Imag5/2 -> tostring8/2(In2)
  Complex to Real-Imag6/1 -> tostring8/3(In3)
  Complex to Real-Imag6/2 -> tostring8/4(In4)
  tostring8/3(Out3) -> Scope6/3
  tostring8/4(Out4) -> Scope6/4
  In1/1 -> Complex to Real-Imag5/1
  In2/1 -> Complex to Real-Imag6/1

== system OFDM0010/Subsystem5/Subsystem4 ==
  Enable : EnablePort
  Frame Status Conversion2 : dspobslib/Frame Status Conversion  SystemSampleTime=-1  growRefPort=off  outframe=Frame-based
  Math Function : Math  Operator=reciprocal  SaturateOnIntegerOverflow=on
  PN Sequence Generator : commseqgen2/PN Sequence Generator  poly=[1 0 0 0 0 1 1]  ini_sta=[0 0 0 0 0 1]  outBitMaskSource=Dialog parameter  shift=0  outVarSiz=off  maxOutSizeMode=Dialog parameter  maxOutSize=[10 1]  Ts=16e-5/2/31  frameBased=on  sampPerFrame=31  reset=off  bitPackedOutputs=off  outDataType=double  numPackedBits=8  bitPackDataSigned=off  bitPackedOutDType=double
  Subsystem23 : Subsystem
  Unipolar to Bipolar Converter : commutil2/Unipolar to Bipolar Converter  SystemSampleTime=-1  M=2  polarity=Positive  dataType=Inherit via internal rule
  Out1 : Outport
  wires:
  PN Sequence Generator/1 -> Unipolar to Bipolar Converter/1
  Frame Status Conversion2/1 -> Out1/1
  Math Function/1 -> Frame Status Conversion2/1, Subsystem23/1(In1)
  Unipolar to Bipolar Converter/1 -> Math Function/1, Subsystem23/2(In2)

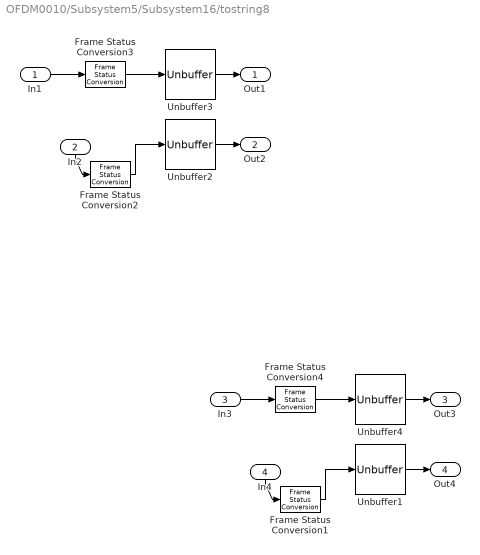
== system OFDM0010/Subsystem5/Subsystem16/tostring8 ==
  In1 : Inport
  In2 : Inport  Port=2
  In3 : Inport  Port=3
  In4 : Inport  Port=4
  Frame Status Conversion{1..4} (4 alike) : dspobslib/Frame Status Conversion  SystemSampleTime=-1  growRefPort=off  outframe=Sample-based
  Unbuffer{1..4} (4 alike) : Unbuffer  SampleBasedProcessing=Same as frame based
  Out1 : Outport
  Out2 : Outport  Port=2
  Out3 : Outport  Port=3
  Out4 : Outport  Port=4
  wires:
  Frame Status Conversion3/1 -> Unbuffer3/1
  Frame Status Conversion2/1 -> Unbuffer2/1
  In1/1 -> Frame Status Conversion3/1
  In2/1 -> Frame Status Conversion2/1
  Unbuffer3/1 -> Out1/1
  Unbuffer2/1 -> Out2/1
  Frame Status Conversion4/1 -> Unbuffer4/1
  Frame Status Conversion1/1 -> Unbuffer1/1
  In3/1 -> Frame Status Conversion4/1
  In4/1 -> Frame Status Conversion1/1
  Unbuffer4/1 -> Out3/1
  Unbuffer1/1 -> Out4/1

== system OFDM0010/Subsystem5/Subsystem4/Subsystem23 ==
  In1 : Inport
  In2 : Inport  Port=2
  Scope : Scope  NumInputPorts=2
      settings: YMin=-5~-5  YMax=5~5
  tostring : Subsystem
  tostring1 : Subsystem
  wires:
  tostring/1(Out1) -> Scope/1
  tostring1/1(Out1) -> Scope/2
  In1/1 -> tostring/1(In1)
  In2/1 -> tostring1/1(In1)

== system OFDM0010/Subsystem5/Subsystem4/Subsystem23/tostring ==
  In1 : Inport
  Frame Status Conversion5 : dspobslib/Frame Status Conversion  SystemSampleTime=-1  growRefPort=off  outframe=Sample-based
  Unbuffer : Unbuffer  SampleBasedProcessing=Same as frame based
  Out1 : Outport
  wires:
  Frame Status Conversion5/1 -> Unbuffer/1
  In1/1 -> Frame Status Conversion5/1
  Unbuffer/1 -> Out1/1

== system OFDM0010/Subsystem5/Subsystem4/Subsystem23/tostring1 ==
  In1 : Inport
  Frame Status Conversion1 : dspobslib/Frame Status Conversion  SystemSampleTime=-1  growRefPort=off  outframe=Sample-based
  Unbuffer1 : Unbuffer  SampleBasedProcessing=Same as frame based
  Out1 : Outport
  wires:
  Frame Status Conversion1/1 -> Unbuffer1/1
  In1/1 -> Frame Status Conversion1/1
  Unbuffer1/1 -> Out1/1
